simulink model "model"  (R2022a)
settings: Solver=FixedStepAuto  StartTime=0.0  StopTime=1e2  RelTol=1e-3
settings Model: Creator=mrem  LastModifiedBy=mrem

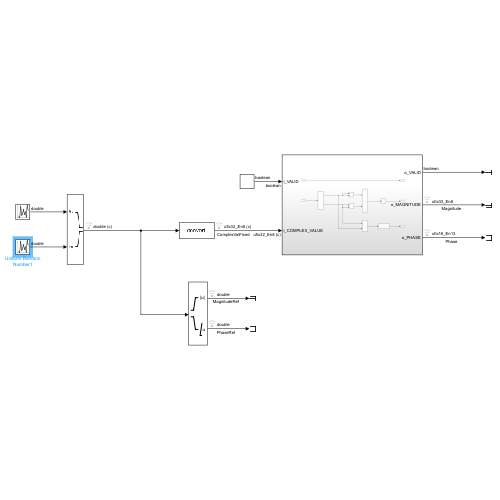
[thumbnail: Simulink's stored preview of the top-level diagram]
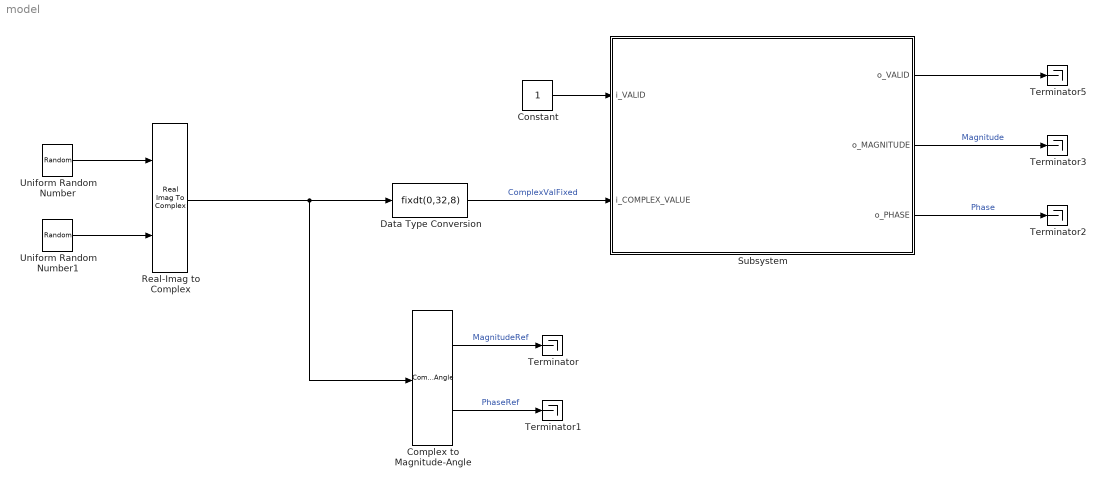
== system model ==
  Complex to Magnitude-Angle : ComplexToMagnitudeAngle
  Constant : Constant  OutDataTypeStr=boolean  SampleTime=-1
  Data Type Conversion : DataTypeConversion  OutDataTypeStr=fixdt(0,32,8)  RndMeth=Round  SaturateOnIntegerOverflow=off
  Real-Imag to Complex : RealImagToComplex
  Subsystem : Subsystem
  Terminator{,1..3,5} (5 alike) : Terminator
  Uniform Random Number : UniformRandomNumber  Minimum=0  Maximum=16777215.9909375  Seed=24  SampleTime=1
  Uniform Random Number1 : UniformRandomNumber  Minimum=0  Maximum=16777215.9909375  Seed=25  SampleTime=1
  wires:
  Constant/1 -> Subsystem/1(i_VALID)
  Uniform Random Number1/1 -> Real-Imag to Complex/2
  Uniform Random Number/1 -> Real-Imag to Complex/1
  Real-Imag to Complex/1 -> Complex to Magnitude-Angle/1, Data Type Conversion/1
  Complex to Magnitude-Angle/1 -> Terminator/1  "MagnitudeRef"
  Complex to Magnitude-Angle/2 -> Terminator1/1  "PhaseRef"
  Subsystem/2(o_MAGNITUDE) -> Terminator3/1  "Magnitude"
  Subsystem/3(o_PHASE) -> Terminator2/1  "Phase"
  Subsystem/1(o_VALID) -> Terminator5/1
  Data Type Conversion/1 -> Subsystem/2(i_COMPLEX_VALUE)  "ComplexValFixed"

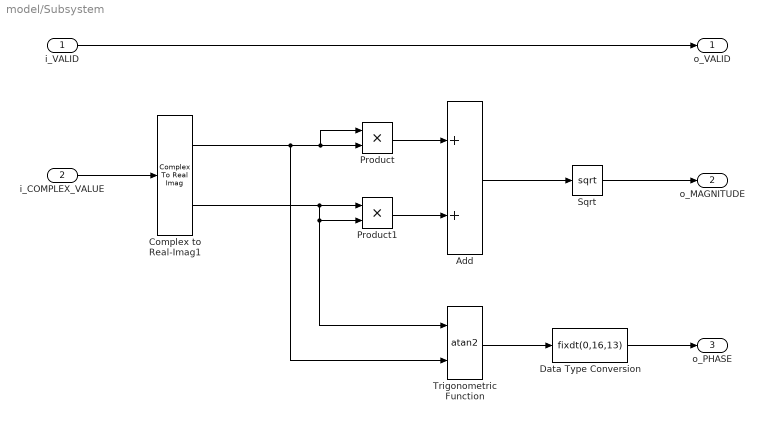
== system model/Subsystem ==
  i_VALID : Inport  OutDataTypeStr=boolean
  i_COMPLEX_VALUE : Inport  Port=2  OutDataTypeStr=fixdt(0,32,8)  LockScale=on
      settings: SignalType=complex
  Add : Sum
  Complex to Real-Imag1 : ComplexToRealImag
  Data Type Conversion : DataTypeConversion  OutDataTypeStr=fixdt(0,16,13)  SaturateOnIntegerOverflow=off  RndMeth=Floor
  Product : Product
  Product1 : Product
  Sqrt : Sqrt  OutDataTypeStr=fixdt(0,33,8)
  Trigonometric Function : Trigonometry  Operator=atan2  ApproximationMethod=CORDIC
  o_VALID : Outport  OutDataTypeStr=boolean
  o_MAGNITUDE : Outport  Port=2
  o_PHASE : Outport  Port=3
  wires:
  i_VALID/1 -> o_VALID/1
  Complex to Real-Imag1/1 -> Trigonometric Function/2, Product/1, Product/2
  i_COMPLEX_VALUE/1 -> Complex to Real-Imag1/1
  Add/1 -> Sqrt/1
  Complex to Real-Imag1/2 -> Trigonometric Function/1, Product1/2, Product1/1
  Sqrt/1 -> o_MAGNITUDE/1
  Product1/1 -> Add/2
  Trigonometric Function/1 -> Data Type Conversion/1
  Product/1 -> Add/1
  Data Type Conversion/1 -> o_PHASE/1
